simulink model "Parallel_OPT"  (R2020a)
settings: Solver=FixedStepAuto  StartTime=0.0  StopTime=10  FixedStep=.01  MaxStep=.01  RelTol=1e-3
InitFcn:
  | Kp = 1;
  | Ki = 1;
  | Kd = 1;
values from neighbouring files (symbols this model uses):
  c = app.cNmradsEditField.Value    [Parallel_OPT_exported.m]
  g = 9.8    [Parallel_OPT_exported.m]
  L = app.LmEditField.Value    [Parallel_OPT_exported.m]
  m = app.massekgEditField.Value    [Parallel_OPT_exported.m]
libraries: simulink_extras x3
settings Model: Creator=hussein  LastModifiedBy=hussein
settings DataIOCC: SaveOutput=off  SignalLogging=off  DSMLogging=off  ReturnWorkspaceOutputs=off

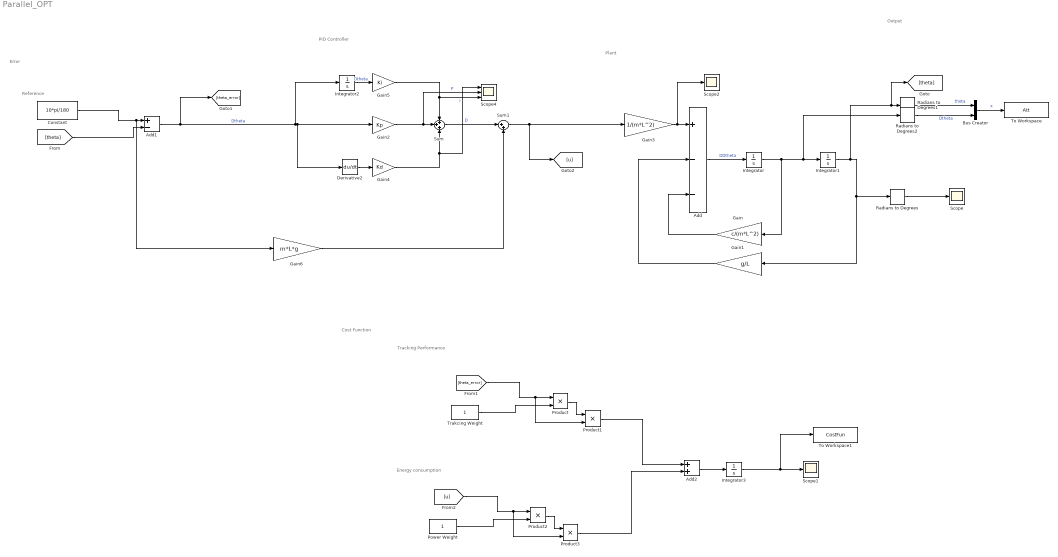
== system Parallel_OPT ==
  note: Cost Function
  note: Tracking Performance
  note: Energy consumption
  note: Output
  note: Plant
  note: Error
  note: Reference
  note: PID Controller
  Add : Sum  Inputs=+--
  Add1 : Sum  Inputs=+-
  Add2 : Sum
  Bus Creator : BusCreator  Inputs=2
  Constant : Constant  Value=10*pi/180
  Derivative2 : Derivative
  Gain : Gain  Gain=c/(m*L^2)
  Gain1 : Gain  Gain=g/L
  Gain2 : Gain  Gain=Kp
  Gain3 : Gain  Gain=1/(m*L^2)
  Gain4 : Gain  Gain=Kd
  Gain5 : Gain  Gain=Ki
  Gain6 : Gain  Gain=m*L*g
  Integrator{,1..3} (4 alike) : Integrator
  Power Weight : Constant
  Product{,1..3} (4 alike) : Product
  Radians to Degrees : simulink_extras/Transformations/Radians to Degrees
  Radians to Degrees1 : simulink_extras/Transformations/Radians to Degrees
  Radians to Degrees2 : simulink_extras/Transformations/Radians to Degrees
  Scope : Scope
  Scope1 : Scope
  Scope2 : Scope
  Scope4 : Scope  NumInputPorts=3
  Sum : Sum  Inputs=+++
  Sum1 : Sum  Inputs=|++
  To Workspace : ToWorkspace  VariableName=Att  SaveFormat=Timeseries  SampleTime=-1
  To Workspace1 : ToWorkspace  VariableName=CostFun  SaveFormat=Timeseries  SampleTime=-1
  Trakcing Weight : Constant
  wires:
  Add/1 -> Integrator/1  "DDtheta"
  Gain/1 -> Add/3
  Gain1/1 -> Add/2
  Gain3/1 -> Scope2/1, Add/1
  Bus Creator/1 -> To Workspace/1  "x"
  Add1/1 -> [theta_error], Integrator2/1, Derivative2/1, Gain2/1  "Dtheta"
  Gain2/1 -> Scope4/2, Sum/2  "P"
  Gain5/1 -> Sum/1, Scope4/3  "I"
  Gain4/1 -> Scope4/1, Sum/3  "D"
  Radians to Degrees/1 -> Scope/1
  [theta] -> Add1/2
  Sum/1 -> Sum1/1
  Integrator2/1 -> Gain5/1  "Dtheta"
  Derivative2/1 -> Gain4/1
  Constant/1 -> Gain6/1, Add1/1
  Gain6/1 -> Sum1/2
  Sum1/1 -> [u], Gain3/1
  Integrator1/1 -> Radians to Degrees1/1, [theta], Gain1/1, Radians to Degrees/1
  Integrator/1 -> Gain/1, Radians to Degrees2/1, Integrator1/1
  Radians to Degrees1/1 -> Bus Creator/1  "theta"
  Radians to Degrees2/1 -> Bus Creator/2  "Dtheta"
  [theta_error] -> Product1/2, Product/1
  Trakcing Weight/1 -> Product/2
  Product/1 -> Product1/1
  Product2/1 -> Product3/1
  Power Weight/1 -> Product2/2
  [u] -> Product2/1, Product3/2
  Product1/1 -> Add2/1
  Product3/1 -> Add2/2
  Add2/1 -> Integrator3/1
  Integrator3/1 -> To Workspace1/1, Scope1/1
